simulink model "Ejer3"  (R2023b)
settings: Solver=VariableStepAuto  StartTime=0.0  StopTime=10.0  RelTol=1e-3
settings Model: Creator=alfre  LastModifiedBy=alfre

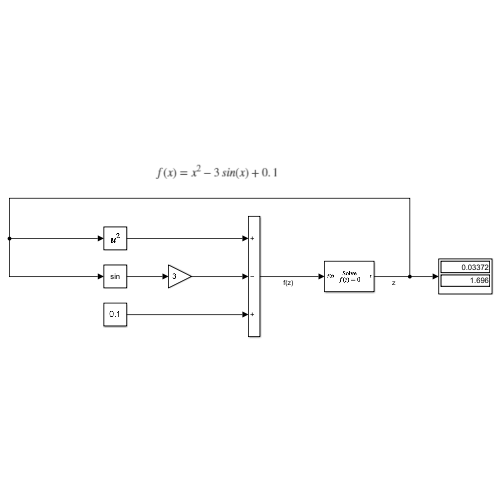
[thumbnail: Simulink's stored preview of the top-level diagram]
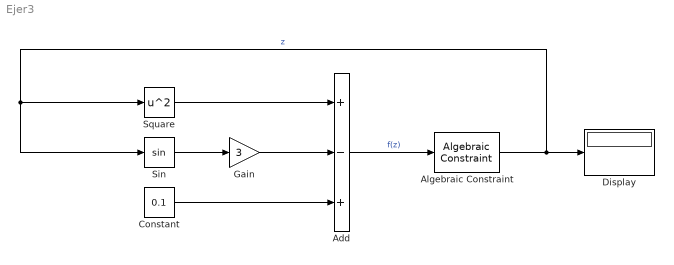
== system Ejer3 ==
  Add : Sum  Inputs=+-+
  Algebraic Constraint : AlgebraicConstraint  InitialGuess=[0.1, 1.5]
  Constant : Constant  Value=0.1
  Display : Display
  Gain : Gain  Gain=3
  Sin : Trigonometry
  Square : Math  Operator=square
  wires:
  Algebraic Constraint/1 -> Square/1, Sin/1, Display/1  "z"
  Square/1 -> Add/1
  Sin/1 -> Gain/1
  Gain/1 -> Add/2
  Add/1 -> Algebraic Constraint/1  "f(z)"
  Constant/1 -> Add/3
